simulink model "WindFarmType4AverageModel"  (R2024b)
settings: Solver=FixedStepDiscrete  StartTime=0.0  StopTime=5  RelTol=1e-4
PreLoadFcn:
  | Ts=50e-6;
InitFcn:
  | xInitial = WindFarmType4AverageModelInit;
  | Ts=50e-6;
undefined symbols (not defined in the file): D1, D11, Delta, DiscIntNeverNeededParam, find_system
libraries: spsSecondOrderFilterLib x54, spsabctodq0Lib x30, spsThreePhaseVIMeasurementLib x26, simulink_extras x24, spsFirstOrderFilterLib x24, spsControlledVoltageSourceLib x18, spsThreePhaseTransformerTwoWindingsLib x14, simulink x12, spsSeriesRLCBranchLib x7, spsThreePhasePISectionLineLib x7, spsThreePhaseSeriesRLCLoadLib x7, spsSynchronousMachinepuStandardLib x7
(part 2 of 14)

== system WindFarmType4AverageModel/Noble Chateaugay (106.5 MW) ==
  230 kV/34.5 kV 47 MVA : spsThreePhaseTransformerTwoWindingsLib/Three-Phase Transformer (Two Windings)  Winding1Connection=Yg  Winding2Connection=Delta (D1)  CoreType=Three single-phase transformers  SetSaturation=off  Hysteresis=off  DataFile='basic_model'  SetInitialFlux=off  Measurements=None  UNITS=pu  NominalPower=[47e6 60 ]  Winding1="[ 230e3  0.08/30   0.08 ]"  Winding2="[34.5e3  0.08/30  0.08]"  Rm=500  Lm=500  L0=0.5  Saturation="[ 0,0  ;  0.005,1.2  ;  1.0,1.4 ]"  InitialFluxes=[ 0.8 , -0.8 , 0.7 ]  BreakLoop=off  DiscreteSolver=Trapezoidal iterative  DataType=off  TransfoNumber=0
  34.5 kV/ 690V 5*2.5 MVA : spsThreePhaseTransformerTwoWindingsLib/Three-Phase Transformer (Two Windings)  Winding1Connection=Delta (D11)  Winding2Connection=Yg  CoreType=Three single-phase transformers  SetSaturation=off  Hysteresis=off  DataFile='hysteresis'  SetInitialFlux=off  Measurements=None  UNITS=pu  NominalPower="[2.5e6*5  60]"  Winding1=[34.5e3 , 0.025/30 , 0.025]  Winding2=[690, 0.025/30 , 0.025]  Rm=500  Lm=inf  L0=0.5  Saturation=[ 0,0 ; 0.0024,1.2 ; 1.0,1.52 ]  InitialFluxes=[ 0.8 , -0.8 , 0.7 ]  BreakLoop=off  DiscreteSolver=Trapezoidal iterative  DataType=off  TransfoNumber=0
  5 km line : spsThreePhasePISectionLineLib/Three-Phase PI Section Line  LConnTagsString=a|b|c  RConnTagsString=A|B|C  Length=5  Frequency=60  Resistances=[0.1153 0.413]  Inductances=[1.05e-3 3.32e-3]  Capacitances=[11.33e-009 5.01e-009]
  B4 (690 V) : spsThreePhaseVIMeasurementLib/Three-Phase V-I Measurement  VoltageMeasurement=phase-to-ground  SetLabelV=on  LabelV=Vabc_B4  Vpu=on  VpuLL=off  CurrentMeasurement=yes  SetLabelI=on  LabelI=Iabc_B4  Ipu=on  Pbase=5*2e6/0.9  Vbase=690  OutputType=Complex  PhasorSimulation=off  PSBequivalent=0
  Bus Selector : BusSelector  OutputSignals=Vdc_V,wr_pu,PQ_pu.P_pu,PQ_pu.Q_pu
  Constant : Constant  Value=15
  Constant1 : Constant  Value=0
  Demux : Demux  Outputs=2
  MW : Gain  Gain=71*1.5/0.9  SaturateOnIntegerOverflow=on  OutDataTypeStr=Inherit: Same as input  ParamDataTypeStr=Inherit: Same as input
  Mux : Mux  Inputs=2
  Wind Farm : Subsystem  LoadFcn=%find_system(gcs,'FollowLinks', 'on', 'LookUnderMasks', 'all');  mask(Wind Turbine: Model 7){Nb_wt=71, ShowParameters=Generator data for 1 wind turbine, nom=[1.5e6/0.9 690 60], Reactances=[ 1.305, 0.296, 0.252, 0.474,  0.243,  0.18 ], Time_constants=[  4.49  0.0681  0.0513  ], Resistance=0.006, mec=[0.62 0.01 1], init=[ 0  0  0  0  0  0  0  0  1 ], Vnom=575, Imax_grid_conv=1.1, RL_grid=[ 0.15 0.15/50], C_var_filter1=150e3, Vdc_nom=1100, C_DClink1=90000e-6, L_R_Boost=[0.0012     5e-3], Pmec1=2e6, wind_speed_CpMax=11, wind0=11, DisplayTurbChar=off, H_WT=4.32, Ksh=0.3, D_mutual=1.5, w_wt0=1, torque0=1, Kdc=[1.1   27.5], Ki_var_reg=0.05, Ki_volt_reg=2, Kgrid_side_cur_reg=[1  50], Kspeed=[5 1], Kboost_cur_reg=[0.025 100], Kp_pitch=15, Kcompensation=[1.5  6], Kfield=[10  20], pitch_max=27, pitch_rate=10, Ts=Ts}
      mask prompts: Nb_wt "Number of wind turbines:"; ShowParameters "Display:"; nom "Nom. power, L-L volt. and freq.: [Pn (VA), Vn (Vrms), fn (Hz)]"; Reactances "Reactances [Xd Xd' Xd'' Xq Xq'' Xl] (p.u.):"; Time_constants "Time constants [Tdo' Tdo'' Tq''] (s):"; Resistance "Resistance Rs (p.u.):"; mec "Inertia constant, friction factor, and pairs of poles: [ H(s)  F(p.u.)  p ]"; init "Initial conditions: [dw(%) th(deg) ia,ib,ic(pu) pha,phb,phc(deg) Vf(pu)]:"; Vnom "Grid-side converter nominal AC voltage (V):"; Imax_grid_conv "Grid-side converter maximum AC current (pu based on generator power and converter nominal AC voltage):"; RL_grid "Grid-side coupling inductor [ L(pu) R(pu),pu based on generator power and converter nominal AC voltage] :"; C_var_filter1 "Line filter capacitor (Q=50) (var):"; Vdc_nom "Nominal DC bus voltage (V)"; C_DClink1 "DC bus capacitor (F):"; L_R_Boost "Boost converter inductance [L(H) R(ohm)]:"; Pmec1 "Nominal mechanical output power (W):"; wind_speed_CpMax "Wind speed at nominal speed and at Cp max (must be between 6 m/s and 30 m/s) (m/s):"; wind0 "Initial wind speed (m/s):"; DisplayTurbChar "Display wind turbine power characteristics:"; H_WT "Wind turbine inertia constant H (s):"; Ksh "Shaft spring constant refer to high-speed shaft (pu of nominal mechanical torque/rad):"; D_mutual "Shaft mutual damping (pu of nominal mechanical torque/pu dw):"; w_wt0 "Turbine initial speed (pu of nominal speed):"; torque0 "Initial output torque (pu of nominal mechanical torque):"; Kdc "DC bus voltage regulator gains [Kp Ki]:"; Ki_var_reg "Grid-side converter var regulator gain [ Ki]:"; Ki_volt_reg "Grid-side converter voltage regulator gain [ Ki]:"; Kgrid_side_cur_reg "Grid-side converter current regulator gains [Kp Ki]:"; Kspeed "Speed regulator gains [Kp Ki]:"; Kboost_cur_reg "Boost inductor current regulator gains [Kp Ki]:"; Kp_pitch "Pitch controller gain [Kp]:"; Kcompensation "Pitch compensation gains [Kp Ki]:"; Kfield "Field excitation gains [Kp Ki]:"; pitch_max "Maximum pitch angle (deg):"; pitch_rate "Maximum rate of change of pitch angle (deg/s)"; Ts "Sample time (s):"
      mask help: This block implements a model of a variable speed pitch controlled wind turbine using a synchronous generator.
      mask init: same as WindFarmType4AverageModel/Jericho Rise (77.7 MW)/Wind Farm
      mask TypeOptions ShowParameters: Generator data for 1 wind turbine | Converters data for 1 wind turbine | Turbine data for 1 wind turbine | Drive train data for 1 wind turbine | Control parameters for 1 wind turbine
      mask Callback ShowParameters:
      | BlockName=getfullname(gcb);
      | %
      | Param_Show=get_param(BlockName,'ShowParameters');
      | Param_DisplayTurbChar=get_param(BlockName,'DisplayTurbChar');
      | 
      | p_mask{3}='off';p_mask{4}='off';p_mask{5}='off';
      | p_mask{6}='off';p_mask{7}='off';p_mask{8}='off';p_mask{9}='off';
      | p_mask{10}='off';p_mask{11}='off';p_mask{12}='off';p_mask{13}='off';
      | p_mask{14}='off';p_mask{15}='off';p_mask{16}='off';p_mask{17}='off';
      | p_mask{18}='off';p_mask{19}='off';p_mask{20}='off';p_mask{21}='off';
      | p_mask{22}='off';p_mask{23}='off';p_mask{24}='off';p_mask{25}='off';
      | p_mask{26}='off';p_mask{27}='off';p_mask{28}='off';p_mask{29}='off';
      | p_mask{30}='off';p_mask{31}='off';p_mask{32}='off';p_mask{33}='off';
      | p_mask{34}='off';p_mask{35}='off';
      | 
      | switch Param_Show
      | 	case 'Generator data for 1 wind turbine'
      | 		p_mask{3}='on';p_mask{4}='on';p_mask{5}='on';
      |         p_mask{6}='on';p_mask{7}='on';p_mask{8}='on';
      |     case 'Converters data for 1 wind turbine'
      | 		p_mask{9}='on';p_mask{10}='on';p_mask{11}='on';
      |         p_mask{12}='on';p_mask{13}='on';p_mask{14}='on';p_mask{15}='on';
      | 	case 'Turbine data for 1 wind turbine'
      | 		p_mask{16}='on';p_mask{17}='on';p_mask{18}='on';p_mask{19}='on';
      |     case 'Drive train data for 1 wind turbine'
      |         p_mask{20}='on';p_mask{21}='on';p_mask{22}='on';p_mask{23}='on';
      |         p_mask{24}='on';
      |     case 'Control parameters for 1 wind turbine'
      |         p_mask{25}='on';p_mask{26}='on';p_mask{27}='on';
      |         p_mask{28}='on';p_mask{29}='on';p_mask{30}='on';p_mask{31}='on';
      |         p_mask{32}='on';p_mask{33}='on';p_mask{34}='on';p_mask{35}='on';
      | end
      | 
      | ParVisible={'on','on',p_mask{3},p_mask{4},p_mask{5},p_mask{6},...
      |     p_mask{7},p_mask{8},p_mask{9},p_mask{10},p_mask{11},p_mask{12},...
      |     p_mask{13},p_mask{14},p_mask{15},p_mask{16},p_mask{17},p_mask{18},...
      |     p_mask{19},p_mask{20},p_mask{21},p_mask{22},p_mask{23},p_mask{24},...
      |     p_mask{25},p_mask{26},p_mask{27},p_mask{28},p_mask{29},p_mask{30},...
      |     p_mask{31},p_mask{32},p_mask{33},p_mask{34},p_mask{35},'on'};
      | %
      | set_param(BlockName,'MaskVisibilities',ParVisible);
      | set_param(BlockName,'DisplayTurbChar',Param_DisplayTurbChar);
      mask Display: disp(' ');
  Wind Farm Scope : Scope  NumInputPorts=6
  A : PMIOPort  Side=Left
  B : PMIOPort  Port=2  Side=Left
  C : PMIOPort  Port=3  Side=Left
  wires:
  Constant1/1 -> Wind Farm/2(Qref_pu)
  [Vabc_B4] -> Wind Farm Scope/1  "Vabc_B575 (pu)"
  Demux/1 -> Wind Farm Scope/5  "P (MW)"
  Bus Selector/1 -> Wind Farm Scope/3  "<Vdc_V>"
  Demux/2 -> Wind Farm Scope/6  "Q (Mvar)"
  Mux/1 -> MW/1
  Bus Selector/2 -> Wind Farm Scope/4  "<wr_pu>"
  Wind Farm/1(m) -> Bus Selector/1
  Bus Selector/3 -> Mux/1  "<P_pu>"
  Bus Selector/4 -> Mux/2  "<Q_pu>"
  MW/1 -> Demux/1
  [Iabc_B4] -> Wind Farm Scope/2  "Iabc_B575 (pu)"
  Constant/1 -> Wind Farm/1("Wind (m/s) ")
  connections:
  B4 (690 V)/LConn2 -- 34.5 kV/ 690V 5*2.5 MVA/RConn2
  B4 (690 V)/RConn1 -- Wind Farm/LConn1
  B4 (690 V)/LConn1 -- 34.5 kV/ 690V 5*2.5 MVA/RConn1
  B4 (690 V)/LConn3 -- 34.5 kV/ 690V 5*2.5 MVA/RConn3
  B4 (690 V)/RConn3 -- Wind Farm/LConn3
  Wind Farm/LConn2 -- B4 (690 V)/RConn2
  5 km line/RConn2 -- 34.5 kV/ 690V 5*2.5 MVA/LConn2
  5 km line/LConn1 -- 230 kV/34.5 kV 47 MVA/RConn1
  C/RConn1 -- 230 kV/34.5 kV 47 MVA/LConn3
  A/RConn1 -- 230 kV/34.5 kV 47 MVA/LConn1
  5 km line/LConn3 -- 230 kV/34.5 kV 47 MVA/RConn3
  5 km line/RConn1 -- 34.5 kV/ 690V 5*2.5 MVA/LConn1
  5 km line/RConn3 -- 34.5 kV/ 690V 5*2.5 MVA/LConn3
  B/RConn1 -- 230 kV/34.5 kV 47 MVA/LConn2
  5 km line/LConn2 -- 230 kV/34.5 kV 47 MVA/RConn2

== system WindFarmType4AverageModel/Noble Clinton (100.5 MW) ==
  230 kV/34.5 kV 47 MVA : spsThreePhaseTransformerTwoWindingsLib/Three-Phase Transformer (Two Windings)  Winding1Connection=Yg  Winding2Connection=Delta (D1)  CoreType=Three single-phase transformers  SetSaturation=off  Hysteresis=off  DataFile='basic_model'  SetInitialFlux=off  Measurements=None  UNITS=pu  NominalPower=[47e6 60 ]  Winding1="[ 230e3  0.08/30   0.08 ]"  Winding2="[34.5e3  0.08/30  0.08]"  Rm=500  Lm=500  L0=0.5  Saturation="[ 0,0  ;  0.005,1.2  ;  1.0,1.4 ]"  InitialFluxes=[ 0.8 , -0.8 , 0.7 ]  BreakLoop=off  DiscreteSolver=Trapezoidal iterative  DataType=off  TransfoNumber=0
  34.5 kV/ 690V 5*2.5 MVA : spsThreePhaseTransformerTwoWindingsLib/Three-Phase Transformer (Two Windings)  Winding1Connection=Delta (D11)  Winding2Connection=Yg  CoreType=Three single-phase transformers  SetSaturation=off  Hysteresis=off  DataFile='hysteresis'  SetInitialFlux=off  Measurements=None  UNITS=pu  NominalPower="[2.5e6*5  60]"  Winding1=[34.5e3 , 0.025/30 , 0.025]  Winding2=[690, 0.025/30 , 0.025]  Rm=500  Lm=inf  L0=0.5  Saturation=[ 0,0 ; 0.0024,1.2 ; 1.0,1.52 ]  InitialFluxes=[ 0.8 , -0.8 , 0.7 ]  BreakLoop=off  DiscreteSolver=Trapezoidal iterative  DataType=off  TransfoNumber=0
  5 km line : spsThreePhasePISectionLineLib/Three-Phase PI Section Line  LConnTagsString=a|b|c  RConnTagsString=A|B|C  Length=5  Frequency=60  Resistances=[0.1153 0.413]  Inductances=[1.05e-3 3.32e-3]  Capacitances=[11.33e-009 5.01e-009]
  B5 (690 V) : spsThreePhaseVIMeasurementLib/Three-Phase V-I Measurement  VoltageMeasurement=phase-to-ground  SetLabelV=on  LabelV=Vabc_B5  Vpu=on  VpuLL=off  CurrentMeasurement=yes  SetLabelI=on  LabelI=Iabc_B5  Ipu=on  Pbase=5*2e6/0.9  Vbase=690  OutputType=Complex  PhasorSimulation=off  PSBequivalent=0
  Bus Selector : BusSelector  OutputSignals=Vdc_V,wr_pu,PQ_pu.P_pu,PQ_pu.Q_pu
  Constant : Constant  Value=15
  Constant1 : Constant  Value=0
  Demux : Demux  Outputs=2
  MW : Gain  Gain=67*1.5/0.9  SaturateOnIntegerOverflow=on  OutDataTypeStr=Inherit: Same as input  ParamDataTypeStr=Inherit: Same as input
  Mux : Mux  Inputs=2
  Wind Farm : Subsystem  LoadFcn=%find_system(gcs,'FollowLinks', 'on', 'LookUnderMasks', 'all');  mask(Wind Turbine: Model 7){Nb_wt=67, ShowParameters=Generator data for 1 wind turbine, nom=[1.5e6/0.9 690 60], Reactances=[ 1.305, 0.296, 0.252, 0.474,  0.243,  0.18 ], Time_constants=[  4.49  0.0681  0.0513  ], Resistance=0.006, mec=[0.62 0.01 1], init=[ 0  0  0  0  0  0  0  0  1 ], Vnom=575, Imax_grid_conv=1.1, RL_grid=[ 0.15 0.15/50], C_var_filter1=150e3, Vdc_nom=1100, C_DClink1=90000e-6, L_R_Boost=[0.0012     5e-3], Pmec1=2e6, wind_speed_CpMax=11, wind0=11, DisplayTurbChar=off, H_WT=4.32, Ksh=0.3, D_mutual=1.5, w_wt0=1, torque0=1, Kdc=[1.1   27.5], Ki_var_reg=0.05, Ki_volt_reg=2, Kgrid_side_cur_reg=[1  50], Kspeed=[5 1], Kboost_cur_reg=[0.025 100], Kp_pitch=15, Kcompensation=[1.5  6], Kfield=[10  20], pitch_max=27, pitch_rate=10, Ts=Ts}
      mask prompts: Nb_wt "Number of wind turbines:"; ShowParameters "Display:"; nom "Nom. power, L-L volt. and freq.: [Pn (VA), Vn (Vrms), fn (Hz)]"; Reactances "Reactances [Xd Xd' Xd'' Xq Xq'' Xl] (p.u.):"; Time_constants "Time constants [Tdo' Tdo'' Tq''] (s):"; Resistance "Resistance Rs (p.u.):"; mec "Inertia constant, friction factor, and pairs of poles: [ H(s)  F(p.u.)  p ]"; init "Initial conditions: [dw(%) th(deg) ia,ib,ic(pu) pha,phb,phc(deg) Vf(pu)]:"; Vnom "Grid-side converter nominal AC voltage (V):"; Imax_grid_conv "Grid-side converter maximum AC current (pu based on generator power and converter nominal AC voltage):"; RL_grid "Grid-side coupling inductor [ L(pu) R(pu),pu based on generator power and converter nominal AC voltage] :"; C_var_filter1 "Line filter capacitor (Q=50) (var):"; Vdc_nom "Nominal DC bus voltage (V)"; C_DClink1 "DC bus capacitor (F):"; L_R_Boost "Boost converter inductance [L(H) R(ohm)]:"; Pmec1 "Nominal mechanical output power (W):"; wind_speed_CpMax "Wind speed at nominal speed and at Cp max (must be between 6 m/s and 30 m/s) (m/s):"; wind0 "Initial wind speed (m/s):"; DisplayTurbChar "Display wind turbine power characteristics:"; H_WT "Wind turbine inertia constant H (s):"; Ksh "Shaft spring constant refer to high-speed shaft (pu of nominal mechanical torque/rad):"; D_mutual "Shaft mutual damping (pu of nominal mechanical torque/pu dw):"; w_wt0 "Turbine initial speed (pu of nominal speed):"; torque0 "Initial output torque (pu of nominal mechanical torque):"; Kdc "DC bus voltage regulator gains [Kp Ki]:"; Ki_var_reg "Grid-side converter var regulator gain [ Ki]:"; Ki_volt_reg "Grid-side converter voltage regulator gain [ Ki]:"; Kgrid_side_cur_reg "Grid-side converter current regulator gains [Kp Ki]:"; Kspeed "Speed regulator gains [Kp Ki]:"; Kboost_cur_reg "Boost inductor current regulator gains [Kp Ki]:"; Kp_pitch "Pitch controller gain [Kp]:"; Kcompensation "Pitch compensation gains [Kp Ki]:"; Kfield "Field excitation gains [Kp Ki]:"; pitch_max "Maximum pitch angle (deg):"; pitch_rate "Maximum rate of change of pitch angle (deg/s)"; Ts "Sample time (s):"
      mask help: This block implements a model of a variable speed pitch controlled wind turbine using a synchronous generator.
      mask init: same as WindFarmType4AverageModel/Jericho Rise (77.7 MW)/Wind Farm
      mask TypeOptions ShowParameters: Generator data for 1 wind turbine | Converters data for 1 wind turbine | Turbine data for 1 wind turbine | Drive train data for 1 wind turbine | Control parameters for 1 wind turbine
      mask Callback ShowParameters:
      | BlockName=getfullname(gcb);
      | %
      | Param_Show=get_param(BlockName,'ShowParameters');
      | Param_DisplayTurbChar=get_param(BlockName,'DisplayTurbChar');
      | 
      | p_mask{3}='off';p_mask{4}='off';p_mask{5}='off';
      | p_mask{6}='off';p_mask{7}='off';p_mask{8}='off';p_mask{9}='off';
      | p_mask{10}='off';p_mask{11}='off';p_mask{12}='off';p_mask{13}='off';
      | p_mask{14}='off';p_mask{15}='off';p_mask{16}='off';p_mask{17}='off';
      | p_mask{18}='off';p_mask{19}='off';p_mask{20}='off';p_mask{21}='off';
      | p_mask{22}='off';p_mask{23}='off';p_mask{24}='off';p_mask{25}='off';
      | p_mask{26}='off';p_mask{27}='off';p_mask{28}='off';p_mask{29}='off';
      | p_mask{30}='off';p_mask{31}='off';p_mask{32}='off';p_mask{33}='off';
      | p_mask{34}='off';p_mask{35}='off';
      | 
      | switch Param_Show
      | 	case 'Generator data for 1 wind turbine'
      | 		p_mask{3}='on';p_mask{4}='on';p_mask{5}='on';
      |         p_mask{6}='on';p_mask{7}='on';p_mask{8}='on';
      |     case 'Converters data for 1 wind turbine'
      | 		p_mask{9}='on';p_mask{10}='on';p_mask{11}='on';
      |         p_mask{12}='on';p_mask{13}='on';p_mask{14}='on';p_mask{15}='on';
      | 	case 'Turbine data for 1 wind turbine'
      | 		p_mask{16}='on';p_mask{17}='on';p_mask{18}='on';p_mask{19}='on';
      |     case 'Drive train data for 1 wind turbine'
      |         p_mask{20}='on';p_mask{21}='on';p_mask{22}='on';p_mask{23}='on';
      |         p_mask{24}='on';
      |     case 'Control parameters for 1 wind turbine'
      |         p_mask{25}='on';p_mask{26}='on';p_mask{27}='on';
      |         p_mask{28}='on';p_mask{29}='on';p_mask{30}='on';p_mask{31}='on';
      |         p_mask{32}='on';p_mask{33}='on';p_mask{34}='on';p_mask{35}='on';
      | end
      | 
      | ParVisible={'on','on',p_mask{3},p_mask{4},p_mask{5},p_mask{6},...
      |     p_mask{7},p_mask{8},p_mask{9},p_mask{10},p_mask{11},p_mask{12},...
      |     p_mask{13},p_mask{14},p_mask{15},p_mask{16},p_mask{17},p_mask{18},...
      |     p_mask{19},p_mask{20},p_mask{21},p_mask{22},p_mask{23},p_mask{24},...
      |     p_mask{25},p_mask{26},p_mask{27},p_mask{28},p_mask{29},p_mask{30},...
      |     p_mask{31},p_mask{32},p_mask{33},p_mask{34},p_mask{35},'on'};
      | %
      | set_param(BlockName,'MaskVisibilities',ParVisible);
      | set_param(BlockName,'DisplayTurbChar',Param_DisplayTurbChar);
      mask Display: disp(' ');
  Wind Farm Scope : Scope  NumInputPorts=6
  A : PMIOPort  Side=Left
  B : PMIOPort  Port=2  Side=Left
  C : PMIOPort  Port=3  Side=Left
  wires:
  Constant1/1 -> Wind Farm/2(Qref_pu)
  [Vabc_B5] -> Wind Farm Scope/1  "Vabc_B575 (pu)"
  Demux/1 -> Wind Farm Scope/5  "P (MW)"
  Bus Selector/1 -> Wind Farm Scope/3  "<Vdc_V>"
  Demux/2 -> Wind Farm Scope/6  "Q (Mvar)"
  Mux/1 -> MW/1
  Bus Selector/2 -> Wind Farm Scope/4  "<wr_pu>"
  Wind Farm/1(m) -> Bus Selector/1
  Bus Selector/3 -> Mux/1  "<P_pu>"
  Bus Selector/4 -> Mux/2  "<Q_pu>"
  MW/1 -> Demux/1
  [Iabc_B5] -> Wind Farm Scope/2  "Iabc_B575 (pu)"
  Constant/1 -> Wind Farm/1("Wind (m/s) ")
  connections:
  B5 (690 V)/LConn2 -- 34.5 kV/ 690V 5*2.5 MVA/RConn2
  B5 (690 V)/RConn1 -- Wind Farm/LConn1
  B5 (690 V)/LConn1 -- 34.5 kV/ 690V 5*2.5 MVA/RConn1
  B5 (690 V)/LConn3 -- 34.5 kV/ 690V 5*2.5 MVA/RConn3
  B5 (690 V)/RConn3 -- Wind Farm/LConn3
  Wind Farm/LConn2 -- B5 (690 V)/RConn2
  5 km line/RConn2 -- 34.5 kV/ 690V 5*2.5 MVA/LConn2
  5 km line/LConn1 -- 230 kV/34.5 kV 47 MVA/RConn1
  230 kV/34.5 kV 47 MVA/LConn3 -- C/RConn1
  230 kV/34.5 kV 47 MVA/LConn1 -- A/RConn1
  5 km line/LConn3 -- 230 kV/34.5 kV 47 MVA/RConn3
  5 km line/RConn1 -- 34.5 kV/ 690V 5*2.5 MVA/LConn1
  5 km line/RConn3 -- 34.5 kV/ 690V 5*2.5 MVA/LConn3
  230 kV/34.5 kV 47 MVA/LConn2 -- B/RConn1
  5 km line/LConn2 -- 230 kV/34.5 kV 47 MVA/RConn2

== system WindFarmType4AverageModel/Noble Ellenburg (81 MW) ==
  230 kV/34.5 kV 47 MVA : spsThreePhaseTransformerTwoWindingsLib/Three-Phase Transformer (Two Windings)  Winding1Connection=Yg  Winding2Connection=Delta (D1)  CoreType=Three single-phase transformers  SetSaturation=off  Hysteresis=off  DataFile='basic_model'  SetInitialFlux=off  Measurements=None  UNITS=pu  NominalPower=[47e6 60 ]  Winding1="[ 230e3  0.08/30   0.08 ]"  Winding2="[34.5e3  0.08/30  0.08]"  Rm=500  Lm=500  L0=0.5  Saturation="[ 0,0  ;  0.005,1.2  ;  1.0,1.4 ]"  InitialFluxes=[ 0.8 , -0.8 , 0.7 ]  BreakLoop=off  DiscreteSolver=Trapezoidal iterative  DataType=off  TransfoNumber=0
  34.5 kV/ 690V 5*2.5 MVA : spsThreePhaseTransformerTwoWindingsLib/Three-Phase Transformer (Two Windings)  Winding1Connection=Delta (D11)  Winding2Connection=Yg  CoreType=Three single-phase transformers  SetSaturation=off  Hysteresis=off  DataFile='hysteresis'  SetInitialFlux=off  Measurements=None  UNITS=pu  NominalPower="[2.5e6*5  60]"  Winding1=[34.5e3 , 0.025/30 , 0.025]  Winding2=[690, 0.025/30 , 0.025]  Rm=500  Lm=inf  L0=0.5  Saturation=[ 0,0 ; 0.0024,1.2 ; 1.0,1.52 ]  InitialFluxes=[ 0.8 , -0.8 , 0.7 ]  BreakLoop=off  DiscreteSolver=Trapezoidal iterative  DataType=off  TransfoNumber=0
  5 km line : spsThreePhasePISectionLineLib/Three-Phase PI Section Line  LConnTagsString=a|b|c  RConnTagsString=A|B|C  Length=5  Frequency=60  Resistances=[0.1153 0.413]  Inductances=[1.05e-3 3.32e-3]  Capacitances=[11.33e-009 5.01e-009]
  B6 (690 V) : spsThreePhaseVIMeasurementLib/Three-Phase V-I Measurement  VoltageMeasurement=phase-to-ground  SetLabelV=on  LabelV=Vabc_B6  Vpu=on  VpuLL=off  CurrentMeasurement=yes  SetLabelI=on  LabelI=Iabc_B6  Ipu=on  Pbase=5*2e6/0.9  Vbase=690  OutputType=Complex  PhasorSimulation=off  PSBequivalent=0
  Bus Selector : BusSelector  OutputSignals=Vdc_V,wr_pu,PQ_pu.P_pu,PQ_pu.Q_pu
  Constant : Constant  Value=15
  Constant1 : Constant  Value=0
  Demux : Demux  Outputs=2
  MW : Gain  Gain=54*1.5/0.9  SaturateOnIntegerOverflow=on  OutDataTypeStr=Inherit: Same as input  ParamDataTypeStr=Inherit: Same as input
  Mux : Mux  Inputs=2
  Wind Farm : Subsystem  LoadFcn=%find_system(gcs,'FollowLinks', 'on', 'LookUnderMasks', 'all');  mask(Wind Turbine: Model 7){Nb_wt=54, ShowParameters=Generator data for 1 wind turbine, nom=[1.5e6/0.9 690 60], Reactances=[ 1.305, 0.296, 0.252, 0.474,  0.243,  0.18 ], Time_constants=[  4.49  0.0681  0.0513  ], Resistance=0.006, mec=[0.62 0.01 1], init=[ 0  0  0  0  0  0  0  0  1 ], Vnom=575, Imax_grid_conv=1.1, RL_grid=[ 0.15 0.15/50], C_var_filter1=150e3, Vdc_nom=1100, C_DClink1=90000e-6, L_R_Boost=[0.0012     5e-3], Pmec1=2e6, wind_speed_CpMax=11, wind0=11, DisplayTurbChar=off, H_WT=4.32, Ksh=0.3, D_mutual=1.5, w_wt0=1, torque0=1, Kdc=[1.1   27.5], Ki_var_reg=0.05, Ki_volt_reg=2, Kgrid_side_cur_reg=[1  50], Kspeed=[5 1], Kboost_cur_reg=[0.025 100], Kp_pitch=15, Kcompensation=[1.5  6], Kfield=[10  20], pitch_max=27, pitch_rate=10, Ts=Ts}
      mask prompts: Nb_wt "Number of wind turbines:"; ShowParameters "Display:"; nom "Nom. power, L-L volt. and freq.: [Pn (VA), Vn (Vrms), fn (Hz)]"; Reactances "Reactances [Xd Xd' Xd'' Xq Xq'' Xl] (p.u.):"; Time_constants "Time constants [Tdo' Tdo'' Tq''] (s):"; Resistance "Resistance Rs (p.u.):"; mec "Inertia constant, friction factor, and pairs of poles: [ H(s)  F(p.u.)  p ]"; init "Initial conditions: [dw(%) th(deg) ia,ib,ic(pu) pha,phb,phc(deg) Vf(pu)]:"; Vnom "Grid-side converter nominal AC voltage (V):"; Imax_grid_conv "Grid-side converter maximum AC current (pu based on generator power and converter nominal AC voltage):"; RL_grid "Grid-side coupling inductor [ L(pu) R(pu),pu based on generator power and converter nominal AC voltage] :"; C_var_filter1 "Line filter capacitor (Q=50) (var):"; Vdc_nom "Nominal DC bus voltage (V)"; C_DClink1 "DC bus capacitor (F):"; L_R_Boost "Boost converter inductance [L(H) R(ohm)]:"; Pmec1 "Nominal mechanical output power (W):"; wind_speed_CpMax "Wind speed at nominal speed and at Cp max (must be between 6 m/s and 30 m/s) (m/s):"; wind0 "Initial wind speed (m/s):"; DisplayTurbChar "Display wind turbine power characteristics:"; H_WT "Wind turbine inertia constant H (s):"; Ksh "Shaft spring constant refer to high-speed shaft (pu of nominal mechanical torque/rad):"; D_mutual "Shaft mutual damping (pu of nominal mechanical torque/pu dw):"; w_wt0 "Turbine initial speed (pu of nominal speed):"; torque0 "Initial output torque (pu of nominal mechanical torque):"; Kdc "DC bus voltage regulator gains [Kp Ki]:"; Ki_var_reg "Grid-side converter var regulator gain [ Ki]:"; Ki_volt_reg "Grid-side converter voltage regulator gain [ Ki]:"; Kgrid_side_cur_reg "Grid-side converter current regulator gains [Kp Ki]:"; Kspeed "Speed regulator gains [Kp Ki]:"; Kboost_cur_reg "Boost inductor current regulator gains [Kp Ki]:"; Kp_pitch "Pitch controller gain [Kp]:"; Kcompensation "Pitch compensation gains [Kp Ki]:"; Kfield "Field excitation gains [Kp Ki]:"; pitch_max "Maximum pitch angle (deg):"; pitch_rate "Maximum rate of change of pitch angle (deg/s)"; Ts "Sample time (s):"
      mask help: This block implements a model of a variable speed pitch controlled wind turbine using a synchronous generator.
      mask init: same as WindFarmType4AverageModel/Jericho Rise (77.7 MW)/Wind Farm
      mask TypeOptions ShowParameters: Generator data for 1 wind turbine | Converters data for 1 wind turbine | Turbine data for 1 wind turbine | Drive train data for 1 wind turbine | Control parameters for 1 wind turbine
      mask Callback ShowParameters:
      | BlockName=getfullname(gcb);
      | %
      | Param_Show=get_param(BlockName,'ShowParameters');
      | Param_DisplayTurbChar=get_param(BlockName,'DisplayTurbChar');
      | 
      | p_mask{3}='off';p_mask{4}='off';p_mask{5}='off';
      | p_mask{6}='off';p_mask{7}='off';p_mask{8}='off';p_mask{9}='off';
      | p_mask{10}='off';p_mask{11}='off';p_mask{12}='off';p_mask{13}='off';
      | p_mask{14}='off';p_mask{15}='off';p_mask{16}='off';p_mask{17}='off';
      | p_mask{18}='off';p_mask{19}='off';p_mask{20}='off';p_mask{21}='off';
      | p_mask{22}='off';p_mask{23}='off';p_mask{24}='off';p_mask{25}='off';
      | p_mask{26}='off';p_mask{27}='off';p_mask{28}='off';p_mask{29}='off';
      | p_mask{30}='off';p_mask{31}='off';p_mask{32}='off';p_mask{33}='off';
      | p_mask{34}='off';p_mask{35}='off';
      | 
      | switch Param_Show
      | 	case 'Generator data for 1 wind turbine'
      | 		p_mask{3}='on';p_mask{4}='on';p_mask{5}='on';
      |         p_mask{6}='on';p_mask{7}='on';p_mask{8}='on';
      |     case 'Converters data for 1 wind turbine'
      | 		p_mask{9}='on';p_mask{10}='on';p_mask{11}='on';
      |         p_mask{12}='on';p_mask{13}='on';p_mask{14}='on';p_mask{15}='on';
      | 	case 'Turbine data for 1 wind turbine'
      | 		p_mask{16}='on';p_mask{17}='on';p_mask{18}='on';p_mask{19}='on';
      |     case 'Drive train data for 1 wind turbine'
      |         p_mask{20}='on';p_mask{21}='on';p_mask{22}='on';p_mask{23}='on';
      |         p_mask{24}='on';
      |     case 'Control parameters for 1 wind turbine'
      |         p_mask{25}='on';p_mask{26}='on';p_mask{27}='on';
      |         p_mask{28}='on';p_mask{29}='on';p_mask{30}='on';p_mask{31}='on';
      |         p_mask{32}='on';p_mask{33}='on';p_mask{34}='on';p_mask{35}='on';
      | end
      | 
      | ParVisible={'on','on',p_mask{3},p_mask{4},p_mask{5},p_mask{6},...
      |     p_mask{7},p_mask{8},p_mask{9},p_mask{10},p_mask{11},p_mask{12},...
      |     p_mask{13},p_mask{14},p_mask{15},p_mask{16},p_mask{17},p_mask{18},...
      |     p_mask{19},p_mask{20},p_mask{21},p_mask{22},p_mask{23},p_mask{24},...
      |     p_mask{25},p_mask{26},p_mask{27},p_mask{28},p_mask{29},p_mask{30},...
      |     p_mask{31},p_mask{32},p_mask{33},p_mask{34},p_mask{35},'on'};
      | %
      | set_param(BlockName,'MaskVisibilities',ParVisible);
      | set_param(BlockName,'DisplayTurbChar',Param_DisplayTurbChar);
      mask Display: disp(' ');
  Wind Farm Scope : Scope  NumInputPorts=6
  A : PMIOPort  Side=Left
  B : PMIOPort  Port=2  Side=Left
  C : PMIOPort  Port=3  Side=Left
  wires:
  Constant1/1 -> Wind Farm/2(Qref_pu)
  [Vabc_B6] -> Wind Farm Scope/1  "Vabc_B575 (pu)"
  Demux/1 -> Wind Farm Scope/5  "P (MW)"
  Bus Selector/1 -> Wind Farm Scope/3  "<Vdc_V>"
  Demux/2 -> Wind Farm Scope/6  "Q (Mvar)"
  Mux/1 -> MW/1
  Bus Selector/2 -> Wind Farm Scope/4  "<wr_pu>"
  Wind Farm/1(m) -> Bus Selector/1
  Bus Selector/3 -> Mux/1  "<P_pu>"
  Bus Selector/4 -> Mux/2  "<Q_pu>"
  MW/1 -> Demux/1
  [Iabc_B6] -> Wind Farm Scope/2  "Iabc_B575 (pu)"
  Constant/1 -> Wind Farm/1("Wind (m/s) ")
  connections:
  B6 (690 V)/LConn2 -- 34.5 kV/ 690V 5*2.5 MVA/RConn2
  B6 (690 V)/RConn1 -- Wind Farm/LConn1
  B6 (690 V)/LConn1 -- 34.5 kV/ 690V 5*2.5 MVA/RConn1
  B6 (690 V)/LConn3 -- 34.5 kV/ 690V 5*2.5 MVA/RConn3
  B6 (690 V)/RConn3 -- Wind Farm/LConn3
  Wind Farm/LConn2 -- B6 (690 V)/RConn2
  34.5 kV/ 690V 5*2.5 MVA/LConn2 -- 5 km line/RConn2
  5 km line/LConn1 -- 230 kV/34.5 kV 47 MVA/RConn1
  C/RConn1 -- 230 kV/34.5 kV 47 MVA/LConn3
  A/RConn1 -- 230 kV/34.5 kV 47 MVA/LConn1
  5 km line/LConn3 -- 230 kV/34.5 kV 47 MVA/RConn3
  34.5 kV/ 690V 5*2.5 MVA/LConn1 -- 5 km line/RConn1
  34.5 kV/ 690V 5*2.5 MVA/LConn3 -- 5 km line/RConn3
  B/RConn1 -- 230 kV/34.5 kV 47 MVA/LConn2
  5 km line/LConn2 -- 230 kV/34.5 kV 47 MVA/RConn2

== system WindFarmType4AverageModel/St. Lawrence-FDR Power Project  ==
  230 kV/20 kV 47 MVA : spsThreePhaseTransformerTwoWindingsLib/Three-Phase Transformer (Two Windings)  Winding1Connection=Yg  Winding2Connection=Delta (D1)  CoreType=Three single-phase transformers  SetSaturation=off  Hysteresis=off  DataFile='basic_model'  SetInitialFlux=off  Measurements=None  UNITS=pu  NominalPower=[47e6 60 ]  Winding1="[ 230e3  0.08/30   0.08 ]"  Winding2="[ 20e3  0.08/30  0.08]"  Rm=500  Lm=500  L0=0.5  Saturation="[ 0,0  ;  0.005,1.2  ;  1.0,1.4 ]"  InitialFluxes=[ 0.8 , -0.8 , 0.7 ]  BreakLoop=off  DiscreteSolver=Trapezoidal iterative  DataType=off  TransfoNumber=0
  Bus Selector : BusSelector  OutputSignals="dq0 components.Stator voltage  vq (pu),dq0 components.Stator voltage  vd (pu),Mechanical.Rotor speed  wm  (pu),Mechanical.Rotor speed deviation  dw (pu),Output active power   Peo (pu)"
  Constant : Constant
  Constant1 : Constant
  Constant2 : Constant  Value=0.75
  Excitation System : spsExcitationSystemLib/Excitation System  tr=20e-3  reg=[ 300, 0.001 ]  exc=[ 1, 0 ]  tgr=[ 0, 0 ]  damp=[ 0.001, 0.1 ]  sat=[ 0, 0 ]  lim=[ -11.5, 11.5, 0 ]  v0="[1.0  1.28]"
  Ground : Ground
  Hydraulic Turbine and Governor : spsHydraulicTurbineandGovernorLib/Hydraulic Turbine and Governor  sm="[ 10/3  0.07 ]"  gate="[  0.01  0.97518  -0.1  0.1 ]"  reg="[  0.05  1.163  0.105  0  0.01  ]"  hyd="[  0  2.67  ]"  dref=0  po=0.7516
  Power Dam Turbine : spsSynchronousMachinepuStandardLib/Synchronous Machine pu Standard  PresetModel=No  MechanicalLoad=Mechanical power Pm  ShowDetailedParameters=on  RotorType=Salient-pole  Units=per unit standard parameters  MeasurementBus=off  NominalParameters=[57e+06 20e+03 60]  Reactances1=[ 1.81, 0.3, 0.23, 1.76, 0.65, 0.25, 0.15 ]  Reactances2=[2.24 0.17 0.12 1.02 0.13 0.08]  dAxisTimeConstants=Short-circuit  qAxisTimeConstants=Short-circuit  TimeConstants1="[ 4.4849  0.0681  0.1  ]"  TimeConstants2=[ 8.0, 0.03, 1.0, 0.07 ]  TimeConstants3="[  4.49  0.0681  0.0513  ]"  TimeConstants4=[ 8.0, 0.03, 0.3371, 0.0295 ]  TimeConstants5=[ 1.01, 0.053, 0.1 ]  TimeConstants6=[ 1.3201, 0.023, 1.0, 0.07 ]  TimeConstants7=[0.012 0.003 0.003]  TimeConstants8=[ 1.3201, 0.0231, 0.3371, 0.0295 ]  StatorResistance=0.037875  Mechanical=[0.1028 0.02056 2]  PolePairs=20  InitialConditions="[ 0  0  0  0  0  0  0  0  1 ]"  SetSaturation=on  Saturation=[0.6404,0.7127,0.8441,0.9214,0.9956,1.082,1.19,1.316,1.457;0.7,0.7698,0.8872,0.9466,0.9969,1.046,1.1,1.151,1.201]  LoadFlowParameters=[1,0,0,0,0]  TsPowergui=0  TsBlock=-1  IterativeModel=Trapezoidal non iterative  IterativeDiscreteModel=Trapezoidal non iterative  BusType=PV  Pref=0  Qref=0  Qmin=-inf  Qmax=inf  PLF=0  QLF=0
  Scope : Scope
  Terminator : Terminator
  Three-Phase Series RLC Load : spsThreePhaseSeriesRLCLoadLib/Three-Phase Series RLC Load  LConnTagsString=A|B|C  Configuration=Y (grounded)  NominalVoltage=1000  Vabc=[1e3 1e3 1e3]  Vabcp=[1e3 1e3 1e3]  NominalFrequency=60  UnbalancedPower=off  ActivePower=100000e3  InductivePower=0  CapacitivePower=0  Pabc=[10e3 9e3 11e3]  QLabc=[100 90 110]  QCabc=[100 90 110]  Pabcp=[10e3 9e3 11e3]  QLabcp=[100 90 110]  QCabcp=[100 90 110]  Measurements=None  LoadType=constant Z
  A : PMIOPort  Side=Left
  B : PMIOPort  Port=2  Side=Left
  C : PMIOPort  Port=3  Side=Left
  wires:
  Excitation System/1 -> Power Dam Turbine/2
  Constant/1 -> Excitation System/1
  Bus Selector/5 -> Hydraulic Turbine and Governor/4  "<Output active power   Peo (pu)>"
  Bus Selector/3 -> Scope/1, Hydraulic Turbine and Governor/3  "<Rotor speed  wm  (pu)>"
  Bus Selector/2 -> Excitation System/2  "<Stator voltage  vd (pu)>"
  Power Dam Turbine/1 -> Bus Selector/1
  Bus Selector/1 -> Excitation System/3  "<Stator voltage  vq (pu)>"
  Hydraulic Turbine and Governor/1 -> Power Dam Turbine/1
  Constant2/1 -> Hydraulic Turbine and Governor/2
  Bus Selector/4 -> Hydraulic Turbine and Governor/5  "<Rotor speed deviation  dw (pu)>"
  Constant1/1 -> Hydraulic Turbine and Governor/1
  Ground/1 -> Excitation System/4
  Hydraulic Turbine and Governor/2 -> Terminator/1
  connections:
  230 kV/20 kV 47 MVA/LConn1 -- A/RConn1
  Power Dam Turbine/RConn2 -- 230 kV/20 kV 47 MVA/RConn2 -- Three-Phase Series RLC Load/LConn2
  Power Dam Turbine/RConn3 -- Three-Phase Series RLC Load/LConn3 -- 230 kV/20 kV 47 MVA/RConn3
  230 kV/20 kV 47 MVA/LConn2 -- B/RConn1
  Power Dam Turbine/RConn1 -- Three-Phase Series RLC Load/LConn1 -- 230 kV/20 kV 47 MVA/RConn1
  230 kV/20 kV 47 MVA/LConn3 -- C/RConn1

== system WindFarmType4AverageModel/Jericho Rise (77.7 MW)/Wind Farm ==
  note: Turbine and Drive Train
  note: Control
  note: Output
  note: Inverter
      | Average Model
  note: DC-DC Boost Converter
      | Average Model
  "Wind (m/s) " : Inport
  Qref_pu : Inport  Port=2
  -> pu : Gain  Gain=1/(Pnom/(3*sqrt(2)/pi*Vnom_gen))  SaturateOnIntegerOverflow=on  OutDataTypeStr=Inherit: Same as input  ParamDataTypeStr=Inherit: Same as input
  Average Switch Voltage : Subsystem
  B_gen : spsThreePhaseVIMeasurementLib/Three-Phase V-I Measurement  VoltageMeasurement=phase-to-phase  SetLabelV=off  LabelV=Vabc  Vpu=on  VpuLL=off  CurrentMeasurement=yes  SetLabelI=off  LabelI=Iabc  Ipu=on  Pbase=Pnom  Vbase=Vnom_gen  OutputType=Complex  PhasorSimulation=off  PSBequivalent=0
  B_grid : spsThreePhaseVIMeasurementLib/Three-Phase V-I Measurement  VoltageMeasurement=phase-to-ground  SetLabelV=off  LabelV=Vabc  Vpu=on  VpuLL=off  CurrentMeasurement=yes  SetLabelI=off  LabelI=Iabc  Ipu=on  Pbase=Pnom  Vbase=Vnom  OutputType=Complex  PhasorSimulation=off  PSBequivalent=0
  B_grid_conv : spsThreePhaseVIMeasurementLib/Three-Phase V-I Measurement  VoltageMeasurement=phase-to-ground  SetLabelV=off  LabelV=Vabc  Vpu=on  VpuLL=off  CurrentMeasurement=no  SetLabelI=off  LabelI=Iabc  Ipu=on  Pbase=Pnom  Vbase=Vnom  OutputType=Complex  PhasorSimulation=off  PSBequivalent=0
  Bus Creator : BusCreator  Inputs=11
  Bus Selector : BusSelector  OutputSignals="Mechanical.Rotor speed  wm  (pu),Mechanical.Rotor mechanical angle  theta (deg)"
  "Choke " : spsThreePhaseSeriesRLCBranchLib/Three-Phase Series RLC Branch  LConnTagsString=A|B|C  RConnTagsString=A|B|C  BranchType=RL  Resistance=R_RL*Vnom^2/Pnom  Inductance=L_RL*Vnom^2/Pnom/(2*pi*Fnom)  Capacitance=[]  Measurements=None
  Control : Subsystem
  Drive Train : Subsystem  mask(Wind Turbine shaft){H_WT=H_WT, Ksh=Ksh, D_mutual=D_mutual, wbase=2*pi*Fnom/p, w_wt0=w_wt0, torque0=torque0, Ts=Ts}
      mask prompts: H_WT "Wind turbine inertia constant H (s):"; Ksh "Shaft spring constant (pu of nominal mechanical torque/rad):"; D_mutual "Shaft mutual damping (pu of nominal mechanical torque/pu dw):"; wbase "Shaft base speed (rad/s):"; w_wt0 "Turbine initial speed (pu of base speed):"; torque0 "Initial output torque (pu of nominal mechanical torque):"; Ts "Sample time (s):"
      mask help:
      | This block implements a wind turbine drive train model. All shaft parameters are referred to high-speed shaft (generator shaft).
      |
      | The first input is the wind turbine torque in per unit (pu) based on the nominal power of the turbine and the base speed of the generator. The second input is the generator speed in pu based on the base speed of the generator.
      |
      | The outputs are:
      | 1- the transmitted torque of the shaft in pu based on the nominal power of the turbine and the base speed of the generator.
      | 2- the wind turbine speed in pu of the base speed of the generator.
  Filter Q=50 : spsThreePhaseSeriesRLCLoadLib/Three-Phase Series RLC Load  LConnTagsString=A|B|C  Configuration=Y (grounded)  NominalVoltage=Vnom  Vabc=[1e3 1e3 1e3]  Vabcp=[1e3 1e3 1e3]  NominalFrequency=Fnom  UnbalancedPower=off  ActivePower=C_var_filter/Q_filter  InductivePower=0  CapacitivePower=C_var_filter  Pabc=[10e3 9e3 11e3]  QLabc=[100 90 110]  QCabc=[100 90 110]  Pabcp=[10e3 9e3 11e3]  QLabcp=[100 90 110]  QCabcp=[100 90 110]  Measurements=None  LoadType=constant Z
  IL : spsCurrentMeasurementLib/Current Measurement  PhasorSimulation=off  OutputType=Complex  PSBequivalent=0
  Inverter and DC-DC Converter Average Models : Subsystem
  Power base for the Generator : Gain  Gain=Pmec/Pnom  SaturateOnIntegerOverflow=on  OutDataTypeStr=Inherit: Same as input  ParamDataTypeStr=Inherit: Same as input
  Product : Product  RndMeth=Zero
  Series RLC Branch1 : spsSeriesRLCBranchLib/Series RLC Branch  LConnTagsString=__new0  RConnTagsString=__new0  BranchType=RL  Resistance=R_Boost  Inductance=L_Boost  SetiL0=off  InitialCurrent=0  Capacitance=1.0  Setx0=off  InitialVoltage=0  Measurements=Branch current
  Synchronous Machine pu Standard : spsSynchronousMachinepuStandardLib/Synchronous Machine pu Standard  PresetModel=No  MechanicalLoad=Mechanical power Pm  ShowDetailedParameters=on  RotorType=Salient-pole  Units=per unit standard parameters  MeasurementBus=off  NominalParameters="[ Pnom  Vnom_gen Fnom ]"  Reactances1=[ 1.81, 0.3, 0.23, 1.76, 0.65, 0.25, 0.15 ]  Reactances2="[ Xd, Xd1, Xd2, Xq,  Xq2,  Xl ]"  dAxisTimeConstants=Open-circuit  qAxisTimeConstants=Short-circuit  TimeConstants1="[ 4.4849  0.0681  0.1  ]"  TimeConstants2=[ 8.0, 0.03, 1.0, 0.07 ]  TimeConstants3="[  Tdo1  Tdo2  Tq2  ]"  TimeConstants4=[ 8.0, 0.03, 0.3371, 0.0295 ]  TimeConstants5=[ 1.01, 0.053, 0.1 ]  TimeConstants6=[ 1.3201, 0.023, 1.0, 0.07 ]  TimeConstants7="[  1.01  0.053  0.051266  ]"  TimeConstants8=[ 1.3201, 0.0231, 0.3371, 0.0295 ]  StatorResistance=Resistance  Mechanical=[ H F p]  PolePairs=1  InitialConditions=init  SetSaturation=off  Saturation=[0.6404,0.7127,0.8441,0.9214,0.9956,1.082,1.19,1.316,1.457;0.7,0.7698,0.8872,0.9466,0.9969,1.046,1.1,1.151,1.201]  LoadFlowParameters=[1,0,0,0,0]  TsPowergui=0  TsBlock=-1  IterativeModel=Trapezoidal non iterative  IterativeDiscreteModel=Trapezoidal non iterative  BusType=PV  Pref=0  Qref=0  Qmin=-inf  Qmax=inf  PLF=0  QLF=0
  Universal Bridge : spsUniversalBridgeLib/Universal Bridge  Arms=3  SnubberResistance=2*Ts_snub/(Pnom/(1000*2*pi*Fnom*Vnom_gen^2))  SnubberCapacitance=Pnom/(1000*2*pi*Fnom*Vnom_gen^2)  Device=Diodes  Ron=1e-6/Nb_wt  Lon=0  ForwardVoltages="[  0  0  ]"  ForwardVoltage=0  GTOparameters=[ 10e-6 , 20e-6 ]  IGBTparameters=[ 1e-6 , 2e-6 ]  Measurements=None  Measurements_2=None  converterType=Rectifier
  V_ab : spsControlledVoltageSourceLib/Controlled Voltage Source  Initialize=on  Source_Type=AC  Amplitude=0  Phase=0  Frequency=0  Measurements=None
  V_bc : spsControlledVoltageSourceLib/Controlled Voltage Source  Initialize=on  Source_Type=AC  Amplitude=0  Phase=0  Frequency=0  Measurements=None
  Wind Turbine : Subsystem  mask(Wind Turbine){Prated=Pmec, c1_c8=c1_c8, K1_K2=K1_K2, wind0=wind0, Ts=Ts}
      mask prompts: Prated "Nominal mechanical output power (W):"; c1_c8 "Coefficients [c1 ... c8]"; K1_K2 "Parameters [K1 K2]"; wind0 "Initial wind speed (m/s):"; Ts "Sample time (s):"
      mask help:
      | This block implements a generic wind turbine models.
      |
      | The first input is the turbine speed in per unit of the generator base speed. For a synchronous or asynchronous generator, the base speed is the synchronous speed. For a permanent-magnet generator, the base speed is defined as the speed producing nominal voltage at  no load. The second input is the blade pitch angle in degrees. The third input is the wind speed in m/s.
      |
      | The output is the torque applied to the drive train in per unit based on the nominal power of the turbine and the base speed of the generator.
      mask init:
      | c1 = c1_c8(1);
      | c2 = c1_c8(2);
      | c3 = c1_c8(3);
      | c4 = c1_c8(4);
      | c5 = c1_c8(5);
      | c6 = c1_c8(6);
      | c7 = c1_c8(7);;
      | c8 = c1_c8(8);
      | 
      | K1=K1_K2(1);
      | K2=K1_K2(2);
      settings: OpenFcn=power_openblockproxy();
      mask Display: disp('');
  deg->rd : Gain  Gain=pi/180  SaturateOnIntegerOverflow=on  OutDataTypeStr=Inherit: Same as input  ParamDataTypeStr=Inherit: Same as input
  A : PMIOPort  Tag=PMCPort  Side=Left
  B : PMIOPort  Tag=PMCPort  Port=2  Side=Left
  C : PMIOPort  Tag=PMCPort  Port=3  Side=Left
  m : Outport  VectorParamsAs1DForOutWhenUnconnected=off
  wires:
  Wind Turbine/1(Tt (pu)) -> Drive Train/1(T_wt (pu))
  [wr] -> Drive Train/2(Generator speed (pu))
  Drive Train/2(T_shaft (pu)) -> Power base for the Generator/1
  Power base for the Generator/1 -> [Tm]
  "Wind (m/s) "/1 -> Wind Turbine/3(Wind speed (m/s))
  Drive Train/1(W_wt (pu)) -> Wind Turbine/1(W_wt (pu))
  [Pitch] -> Wind Turbine/2(Pitch angle (deg))
  Bus Selector/2 -> deg->rd/1  "<Rotor mechanical angle  theta (deg)>"
  deg->rd/1 -> [angle_rotor]
  Bus Selector/1 -> [wr]  "<Rotor speed  wm  (pu)>"
  [wr] -> Product/1
  Synchronous Machine pu Standard/1 -> Bus Selector/1
  B_grid_conv/1 -> [Vabc_grid_conv]
  [Vabc_LL_stator] -> Bus Creator/1  "Vabc_stator_pu"
  [Iabc_stator] -> Bus Creator/2  "Iabc_stator_pu"
  [Vabc_grid] -> Bus Creator/3  "Vabc_grid_pu"
  Bus Creator/1 -> m/1
  [Vabc_grid_conv] -> Bus Creator/4  "Vabc_grid_conv_pu"
  [Iabc_grid_conv] -> Bus Creator/5  "Iabc_grid_conv_pu"
  [Vf] -> Bus Creator/6  "Vfield_pu"
  [wr] -> Bus Creator/7  "wr_pu"
  [Pm_gen] -> Bus Creator/8  "Pm_gen_pu"
  [Pitch] -> Bus Creator/9  "Pitch_deg"
  [Vdc] -> Bus Creator/10  "Vdc_V"
  [Tm] -> Product/2
  Product/1 -> Synchronous Machine pu Standard/1, [Pm_gen]
  [Iabc_grid_conv] -> Inverter and DC-DC Converter Average Models/2(Iabc_grid_conv)
  Inverter and DC-DC Converter Average Models/3(Vswitch (V)) -> Average Switch Voltage/1(Vswitch)
  IL/1 -> -> pu/1
  [IL] -> Inverter and DC-DC Converter Average Models/1(IL)
  B_grid/1 -> [Vabc_grid]
  B_grid/2 -> [Iabc_grid_conv]
  B_gen/1 -> [Vabc_LL_stator]
  B_gen/2 -> [Iabc_stator]
  [Vabc_grid] -> Control/1(Vabc_grid)
  [Iabc_grid_conv] -> Control/2(Iabc_grid_conv)
  [Vabc_LL_stator] -> Control/3(Vabc_LL_stator)
  [Iabc_stator] -> Control/4(Iabc_stator)
  [Vdc] -> Control/6(Vdc)
  Qref_pu/1 -> Control/7(Qref)
  [angle_rotor] -> Control/8(angle_rotor)
  [wr] -> Control/9(wr)
  Control/1(Uctrl_inverter) -> Inverter and DC-DC Converter Average Models/3(Uctrl_inverter)
  Control/2(Duty_Cycle) -> Inverter and DC-DC Converter Average Models/4(Duty_Cycle)  "Duty_cycle"
  Control/3(Pitch_angle) -> [Pitch]
  Control/4(Vf) -> [Vf]
  Inverter and DC-DC Converter Average Models/4(Vdc (V)) -> [Vdc]
  [Vf] -> Synchronous Machine pu Standard/2
  Inverter and DC-DC Converter Average Models/1(Vab (V)) -> V_ab/1
  Inverter and DC-DC Converter Average Models/2(Vbc (V)) -> V_bc/1
  Control/5(PQ_pu) -> [PQ_pu]
  [PQ_pu] -> Bus Creator/11  "PQ_pu"
  [IL] -> Control/5(IL)
  -> pu/1 -> [IL]
  connections:
  B_gen/RConn1 -- Synchronous Machine pu Standard/RConn1
  B_gen/RConn2 -- Synchronous Machine pu Standard/RConn2
  B_gen/RConn3 -- Synchronous Machine pu Standard/RConn3
  B_grid/RConn1 -- "Choke "/LConn1
  B_grid/RConn2 -- "Choke "/LConn2
  B_grid/RConn3 -- "Choke "/LConn3
  B_grid/LConn1 -- A/RConn1 -- Filter Q=50/LConn1
  B/RConn1 -- B_grid/LConn2 -- Filter Q=50/LConn2
  C/RConn1 -- B_grid/LConn3 -- Filter Q=50/LConn3
  "Choke "/RConn1 -- B_grid_conv/LConn1
  "Choke "/RConn2 -- B_grid_conv/LConn2
  "Choke "/RConn3 -- B_grid_conv/LConn3
  Series RLC Branch1/LConn1 -- Universal Bridge/RConn1
  Average Switch Voltage/LConn1 -- Universal Bridge/RConn2
  V_ab/RConn1 -- B_grid_conv/RConn1
  B_grid_conv/RConn3 -- V_bc/LConn1
  V_bc/RConn1 -- V_ab/LConn1 -- B_grid_conv/RConn2
  Universal Bridge/LConn1 -- B_gen/LConn1
  Universal Bridge/LConn2 -- B_gen/LConn2
  Universal Bridge/LConn3 -- B_gen/LConn3
  Series RLC Branch1/RConn1 -- IL/LConn1
  Average Switch Voltage/RConn1 -- IL/RConn1
